simulink model "Bandpass"  (R2013a)
settings: Solver=ode45  StartTime=0.0  StopTime=inf  RelTol=1e-3
libraries: dspsrcs4 x3, dsparch4 x1, simulink_extras x1
settings Model: Creator=MrBigBear  LastModifiedBy=MrBigBear

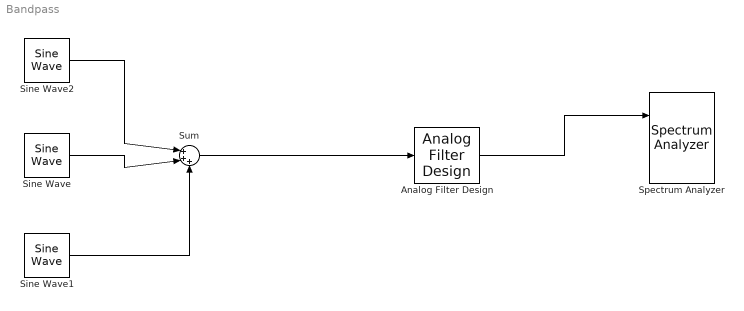
== system Bandpass ==
  Analog Filter Design : dsparch4/Analog Filter Design  method=Butterworth  filttype=Bandpass  N=8  Wlo=2*pi*39000  Whi=2*pi*42000  Rp=2  Rs=40
  Sine Wave : dspsrcs4/Sine Wave  Amplitude=2  Frequency=40000  Phase=0  SampleMode=Continuous  OutComplex=Real  CompMethod=Trigonometric fcn  TableSize=Speed  SampleTime=1/100000000  SamplesPerFrame=1000  ResetState=Restart at time zero  dataType=double  wordLen=16  udDataType=sfix(16)  fracBitsMode=Best precision  numFracBits=15  OutDataTypeStr=double  LastOutDataTypeStr=double
  Sine Wave1 : dspsrcs4/Sine Wave  Amplitude=1  Frequency=24000  Phase=0  SampleMode=Continuous  OutComplex=Real  CompMethod=Trigonometric fcn  TableSize=Speed  SampleTime=1/100000000  SamplesPerFrame=1000  ResetState=Restart at time zero  dataType=double  wordLen=16  udDataType=sfix(16)  fracBitsMode=Best precision  numFracBits=15  OutDataTypeStr=double  LastOutDataTypeStr=double
  Sine Wave2 : dspsrcs4/Sine Wave  Amplitude=0.5  Frequency=80000  Phase=0  SampleMode=Continuous  OutComplex=Real  CompMethod=Trigonometric fcn  TableSize=Speed  SampleTime=1/100000000  SamplesPerFrame=1000  ResetState=Restart at time zero  dataType=double  wordLen=16  udDataType=sfix(16)  fracBitsMode=Best precision  numFracBits=15  OutDataTypeStr=double  LastOutDataTypeStr=double
  Spectrum Analyzer : simulink_extras/Additional Sinks/Spectrum Analyzer  npts=256  fftpts=1024  HowOften=64  sampleT=1E-9
  Sum : Sum  Inputs=|+++
  wires:
  Sine Wave2/1 -> Sum/1
  Sine Wave/1 -> Sum/2
  Sine Wave1/1 -> Sum/3
  Sum/1 -> Analog Filter Design/1
  Analog Filter Design/1 -> Spectrum Analyzer/1
